simulink model "NoThermalControl"  (R2026b)
settings Model: Creator=The MathWorks, Inc.  LastModifiedBy=The MathWorks, Inc.

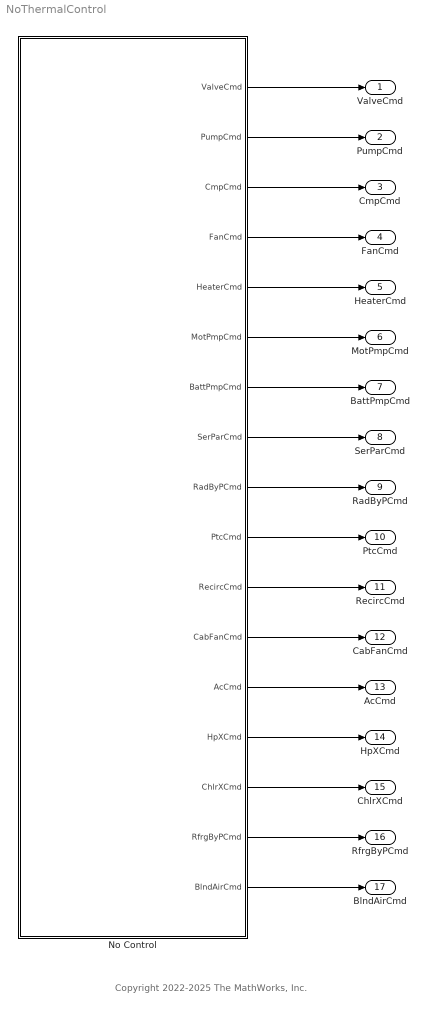
== system NoThermalControl ==
  note: Copyright 2022-2025 The MathWorks, Inc.
  No Control : Subsystem  VariantControl=No Control
  ValveCmd : Outport
  PumpCmd : Outport  Port=2
  CmpCmd : Outport  Port=3
  FanCmd : Outport  Port=4
  HeaterCmd : Outport  Port=5
  MotPmpCmd : Outport  Port=6
  BattPmpCmd : Outport  Port=7
  SerParCmd : Outport  Port=8
  RadByPCmd : Outport  Port=9
  PtcCmd : Outport  Port=10
  RecircCmd : Outport  Port=11
  CabFanCmd : Outport  Port=12
  AcCmd : Outport  Port=13
  HpXCmd : Outport  Port=14
  ChlrXCmd : Outport  Port=15
  RfrgByPCmd : Outport  Port=16
  BlndAirCmd : Outport  Port=17
  wires:
  No Control/1(ValveCmd) -> ValveCmd/1
  No Control/2(PumpCmd) -> PumpCmd/1
  No Control/3(CmpCmd) -> CmpCmd/1
  No Control/4(FanCmd) -> FanCmd/1
  No Control/5(HeaterCmd) -> HeaterCmd/1
  No Control/6(MotPmpCmd) -> MotPmpCmd/1
  No Control/7(BattPmpCmd) -> BattPmpCmd/1
  No Control/8(SerParCmd) -> SerParCmd/1
  No Control/9(RadByPCmd) -> RadByPCmd/1
  No Control/10(PtcCmd) -> PtcCmd/1
  No Control/11(RecircCmd) -> RecircCmd/1
  No Control/12(CabFanCmd) -> CabFanCmd/1
  No Control/13(AcCmd) -> AcCmd/1
  No Control/14(HpXCmd) -> HpXCmd/1
  No Control/15(ChlrXCmd) -> ChlrXCmd/1
  No Control/16(RfrgByPCmd) -> RfrgByPCmd/1
  No Control/17(BlndAirCmd) -> BlndAirCmd/1

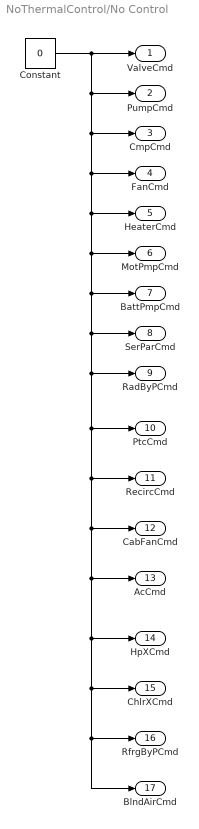
== system NoThermalControl/No Control ==
  Constant : Constant  Value=0  SampleTime=-1
  ValveCmd : Outport
  PumpCmd : Outport  Port=2
  CmpCmd : Outport  Port=3
  FanCmd : Outport  Port=4
  HeaterCmd : Outport  Port=5
  MotPmpCmd : Outport  Port=6
  BattPmpCmd : Outport  Port=7
  SerParCmd : Outport  Port=8
  RadByPCmd : Outport  Port=9
  PtcCmd : Outport  Port=10
  RecircCmd : Outport  Port=11
  CabFanCmd : Outport  Port=12
  AcCmd : Outport  Port=13
  HpXCmd : Outport  Port=14
  ChlrXCmd : Outport  Port=15
  RfrgByPCmd : Outport  Port=16
  BlndAirCmd : Outport  Port=17
  wires:
  Constant/1 -> ValveCmd/1, BlndAirCmd/1, RfrgByPCmd/1, ChlrXCmd/1, HpXCmd/1, AcCmd/1, CabFanCmd/1, RecircCmd/1, PtcCmd/1, RadByPCmd/1, SerParCmd/1, BattPmpCmd/1, MotPmpCmd/1, HeaterCmd/1, FanCmd/1, CmpCmd/1, PumpCmd/1
